simulink model "SingalDispaly"  (R2019b)
settings: Solver=VariableStepAuto  StartTime=0.0  StopTime=Tfinal  RelTol=1e-3
settings Model: EnablePacing=on  PacingRate=0.100000  Creator=Eduardo  LastModifiedBy=Eduardo

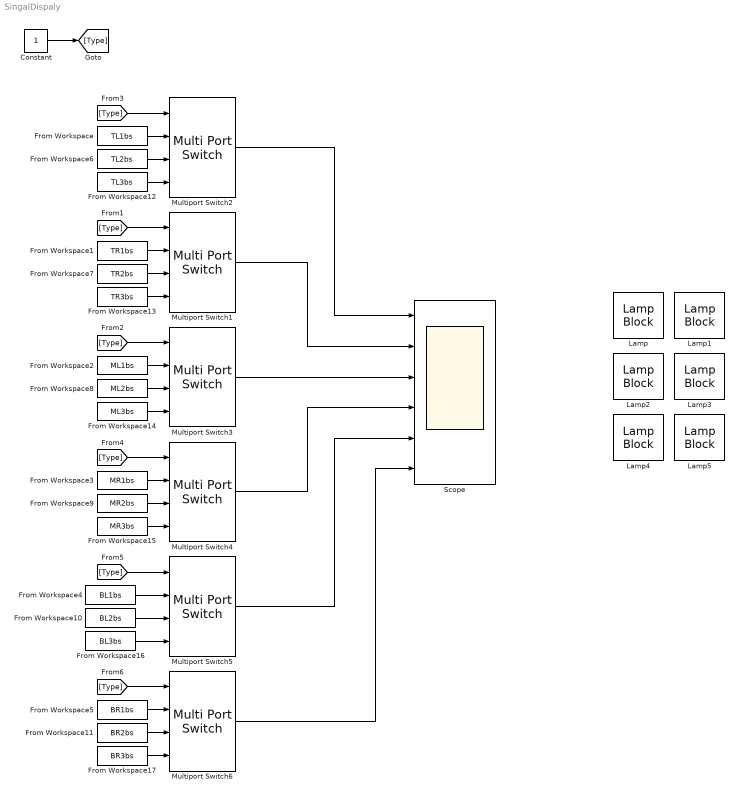
== system SingalDispaly ==
  Constant : Constant
  From Workspace : FromWorkspace  VariableName=TL1bs  SampleTime=0
  From Workspace1 : FromWorkspace  VariableName=TR1bs  SampleTime=0
  From Workspace10 : FromWorkspace  VariableName=BL2bs  SampleTime=0
  From Workspace11 : FromWorkspace  VariableName=BR2bs  SampleTime=0
  From Workspace12 : FromWorkspace  VariableName=TL3bs  SampleTime=0
  From Workspace13 : FromWorkspace  VariableName=TR3bs  SampleTime=0
  From Workspace14 : FromWorkspace  VariableName=ML3bs  SampleTime=0
  From Workspace15 : FromWorkspace  VariableName=MR3bs  SampleTime=0
  From Workspace16 : FromWorkspace  VariableName=BL3bs  SampleTime=0
  From Workspace17 : FromWorkspace  VariableName=BR3bs  SampleTime=0
  From Workspace2 : FromWorkspace  VariableName=ML1bs  SampleTime=0
  From Workspace3 : FromWorkspace  VariableName=MR1bs  SampleTime=0
  From Workspace4 : FromWorkspace  VariableName=BL1bs  SampleTime=0
  From Workspace5 : FromWorkspace  VariableName=BR1bs  SampleTime=0
  From Workspace6 : FromWorkspace  VariableName=TL2bs  SampleTime=0
  From Workspace7 : FromWorkspace  VariableName=TR2bs  SampleTime=0
  From Workspace8 : FromWorkspace  VariableName=ML2bs  SampleTime=0
  From Workspace9 : FromWorkspace  VariableName=MR2bs  SampleTime=0
  Lamp{,1..5} (6 alike) : LampBlock  LabelPosition=Hide
  Multiport Switch{1..6} (6 alike) : MultiPortSwitch
  Scope : Scope  NumInputPorts=6
  wires:
  [Type] -> Multiport Switch2/1
  Constant/1 -> [Type]
  [Type] -> Multiport Switch1/1
  From Workspace/1 -> Multiport Switch2/2
  From Workspace1/1 -> Multiport Switch1/2
  From Workspace6/1 -> Multiport Switch2/3
  From Workspace12/1 -> Multiport Switch2/4
  From Workspace7/1 -> Multiport Switch1/3
  From Workspace13/1 -> Multiport Switch1/4
  [Type] -> Multiport Switch3/1
  From Workspace2/1 -> Multiport Switch3/2
  From Workspace8/1 -> Multiport Switch3/3
  From Workspace14/1 -> Multiport Switch3/4
  [Type] -> Multiport Switch4/1
  From Workspace3/1 -> Multiport Switch4/2
  From Workspace9/1 -> Multiport Switch4/3
  From Workspace15/1 -> Multiport Switch4/4
  [Type] -> Multiport Switch5/1
  From Workspace4/1 -> Multiport Switch5/2
  From Workspace10/1 -> Multiport Switch5/3
  From Workspace16/1 -> Multiport Switch5/4
  [Type] -> Multiport Switch6/1
  From Workspace5/1 -> Multiport Switch6/2
  From Workspace11/1 -> Multiport Switch6/3
  From Workspace17/1 -> Multiport Switch6/4
  Multiport Switch2/1 -> Scope/1
  Multiport Switch1/1 -> Scope/2
  Multiport Switch3/1 -> Scope/3
  Multiport Switch4/1 -> Scope/4
  Multiport Switch5/1 -> Scope/5
  Multiport Switch6/1 -> Scope/6
